simulink model "GearAssembly"  (R2021b)
settings: Solver=VariableStepAuto  StartTime=0.0  StopTime=10.0  RelTol=1e-3
undefined symbols (not defined in the file): GearStateEnum
libraries: LatchUtilities x2
settings Model: Creator=david  LastModifiedBy=david

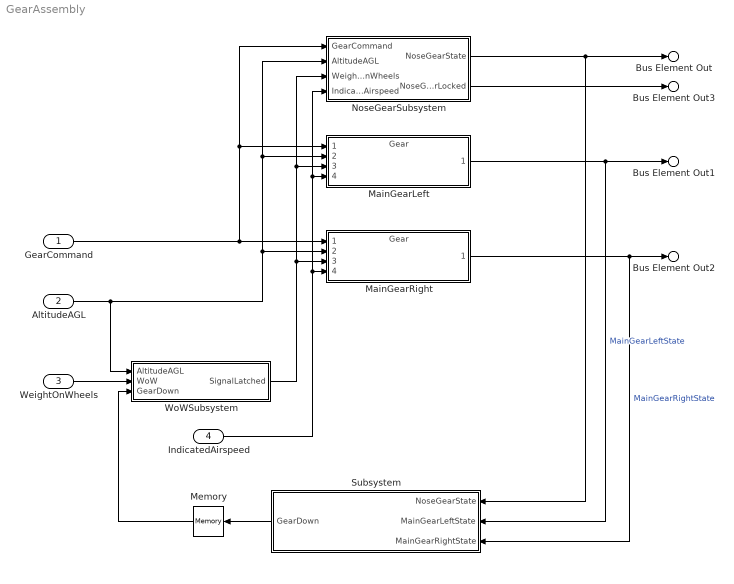
== system GearAssembly ==
  GearCommand : Inport
  AltitudeAGL : Inport  Port=2
  WeightOnWheels : Inport  Port=3
  IndicatedAirspeed : Inport  Port=4  OutDataTypeStr=double  Unit=ft/s
  MainGearLeft : ModelReference  ModelNameDialog=Gear  SimulationMode=Normal  ModelReferenceVersion=1.22
  MainGearRight : ModelReference  ModelNameDialog=Gear  SimulationMode=Normal  ModelReferenceVersion=1.22
  Memory : Memory  InitialCondition=true  InheritSampleTime=on
  NoseGearSubsystem : Subsystem
  Subsystem : Subsystem
  WoWSubsystem : Subsystem
  Bus Element Out : Outport  PortName=GearState  Element=NoseGear
  Bus Element Out1 : Outport  PortName=GearState  Element=MainGearLeft
  Bus Element Out2 : Outport  PortName=GearState  Element=MainGearRignt
  Bus Element Out3 : Outport  PortName=GearState  Element=Locked
  wires:
  AltitudeAGL/1 -> MainGearRight/2, NoseGearSubsystem/2(AltitudeAGL), MainGearLeft/2, WoWSubsystem/1(AltitudeAGL)
  GearCommand/1 -> MainGearRight/1, NoseGearSubsystem/1(GearCommand), MainGearLeft/1
  MainGearLeft/1 -> Bus Element Out1/1, Subsystem/2(MainGearLeftState)  "MainGearLeftState"
  MainGearRight/1 -> Bus Element Out2/1, Subsystem/3(MainGearRightState)  "MainGearRightState"
  IndicatedAirspeed/1 -> MainGearRight/4, NoseGearSubsystem/4(IndicatedAirspeed), MainGearLeft/4
  WoWSubsystem/1(SignalLatched) -> MainGearRight/3, NoseGearSubsystem/3(WeightOnWheels), MainGearLeft/3
  WeightOnWheels/1 -> WoWSubsystem/2(WoW)
  Subsystem/1(GearDown) -> Memory/1
  Memory/1 -> WoWSubsystem/3(GearDown)
  NoseGearSubsystem/1(NoseGearState) -> Subsystem/1(NoseGearState), Bus Element Out/1
  NoseGearSubsystem/2(NoseGearLocked) -> Bus Element Out3/1

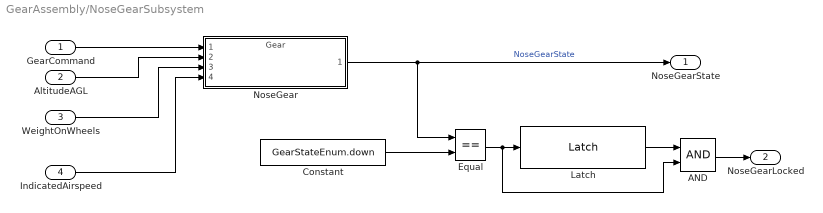
== system GearAssembly/NoseGearSubsystem ==
  GearCommand : Inport
  AltitudeAGL : Inport  Port=2
  WeightOnWheels : Inport  Port=3
  IndicatedAirspeed : Inport  Port=4
  AND : Logic  AllPortsSameDT=off  OutDataTypeStr=boolean
  Constant : Constant  Value=GearStateEnum.down
  Equal : RelationalOperator  Operator===  OutDataTypeStr=boolean  RndMeth=Simplest
  Latch : LatchUtilities/Latch  LatchTime=3
  NoseGear : ModelReference  ModelNameDialog=Gear  SimulationMode=Normal  ModelReferenceVersion=1.22
  NoseGearState : Outport
  NoseGearLocked : Outport  Port=2
  wires:
  WeightOnWheels/1 -> NoseGear/3
  GearCommand/1 -> NoseGear/1
  AltitudeAGL/1 -> NoseGear/2
  IndicatedAirspeed/1 -> NoseGear/4
  Constant/1 -> Equal/2
  NoseGear/1 -> NoseGearState/1, Equal/1  "NoseGearState"
  AND/1 -> NoseGearLocked/1
  Latch/1 -> AND/1
  Equal/1 -> AND/2, Latch/1

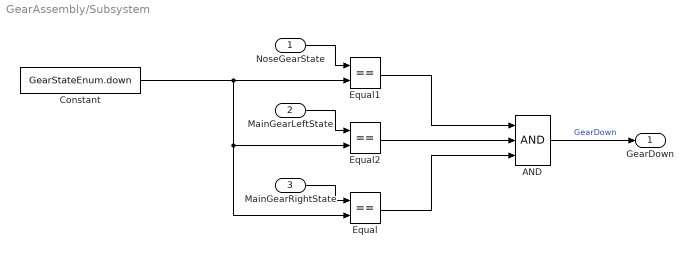
== system GearAssembly/Subsystem ==
  NoseGearState : Inport
  MainGearLeftState : Inport  Port=2
  MainGearRightState : Inport  Port=3
  AND : Logic  Inputs=3  AllPortsSameDT=off  OutDataTypeStr=boolean
  Constant : Constant  Value=GearStateEnum.down
  Equal : RelationalOperator  Operator===  OutDataTypeStr=boolean  RndMeth=Simplest
  Equal1 : RelationalOperator  Operator===  OutDataTypeStr=boolean  RndMeth=Simplest
  Equal2 : RelationalOperator  Operator===  OutDataTypeStr=boolean  RndMeth=Simplest
  GearDown : Outport
  wires:
  AND/1 -> GearDown/1  "GearDown"
  Constant/1 -> Equal/2, Equal2/2, Equal1/2
  Equal1/1 -> AND/1
  Equal2/1 -> AND/2
  Equal/1 -> AND/3
  NoseGearState/1 -> Equal1/1
  MainGearLeftState/1 -> Equal2/1
  MainGearRightState/1 -> Equal/1

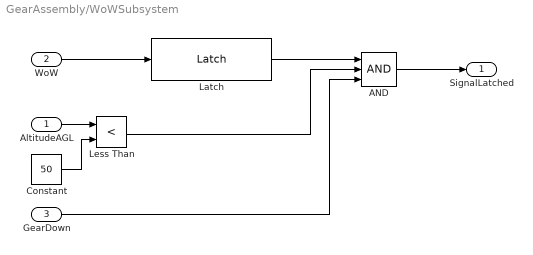
== system GearAssembly/WoWSubsystem ==
  AltitudeAGL : Inport
  WoW : Inport  Port=2
  GearDown : Inport  Port=3
  AND : Logic  Inputs=3  AllPortsSameDT=off  OutDataTypeStr=boolean
  Constant : Constant  Value=50
  Latch : LatchUtilities/Latch  LatchTime=3
  Less Than : RelationalOperator  Operator=<  OutDataTypeStr=boolean  RndMeth=Simplest
  SignalLatched : Outport
  wires:
  Latch/1 -> AND/1
  AltitudeAGL/1 -> Less Than/1
  WoW/1 -> Latch/1
  Constant/1 -> Less Than/2
  Less Than/1 -> AND/2
  GearDown/1 -> AND/3
  AND/1 -> SignalLatched/1
